simulink model "single_joint_controller_only"  (R2023b)
settings: Solver=FixedStepDiscrete  StartTime=0.0  StopTime=1.0  FixedStep=0.001  RelTol=1e-3
settings Model: Creator=user  LastModifiedBy=user
settings HardwareCC: ProdBitPerLong=64  ProdHWDeviceType=Intel->x86-64 (Linux 64)  TargetBitPerLong=64  TargetBitPerPointer=64  TargetBitPerSizeT=64  TargetBitPerPtrDiffT=64  TargetLargestAtomicFloat=Float  TargetIntDivRoundTo=Zero  TargetEndianess=LittleEndian  TargetWordSize=64  TargetHWDeviceType=Intel->x86-64 (Linux 64)  ProdEqTarget=off
settings RTWCC: GenerateReport=on

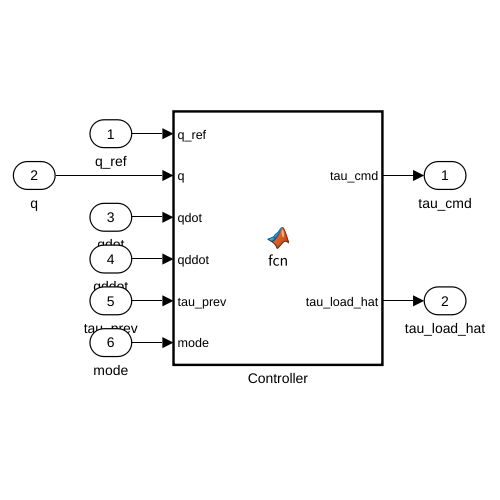
[thumbnail: Simulink's stored preview of the top-level diagram]
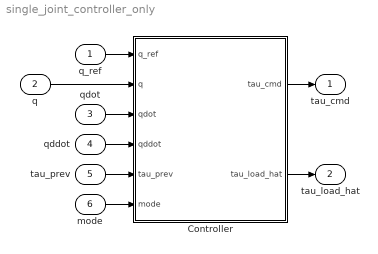
== system single_joint_controller_only ==
  q_ref : Inport  OutDataTypeStr=T_angle
  q : Inport  Port=2  OutDataTypeStr=T_angle
  qdot : Inport  Port=3  OutDataTypeStr=T_speed
  qddot : Inport  Port=4  OutDataTypeStr=T_accel
  tau_prev : Inport  Port=5  OutDataTypeStr=T_torque_wide
  mode : Inport  Port=6  OutDataTypeStr=uint8
  Controller : MATLAB Function  TreatAsAtomicUnit=on  RTWFcnName=usr_pid  RTWFileName=usr_pid
      settings: RTWFileNameOpts=User specified
  tau_cmd : Outport  OutDataTypeStr=T_torque
  tau_load_hat : Outport  Port=2  OutDataTypeStr=T_torque
  wires:
  q_ref/1 -> Controller/1(q_ref)
  q/1 -> Controller/2(q)
  qdot/1 -> Controller/3(qdot)
  qddot/1 -> Controller/4(qddot)
  tau_prev/1 -> Controller/5(tau_prev)
  mode/1 -> Controller/6(mode)
  Controller/1(tau_cmd) -> tau_cmd/1
  Controller/2(tau_load_hat) -> tau_load_hat/1

== matlab function single_joint_controller_only/Controller ==
  data: q_ref input; tau_cmd output; q input; qdot input; qddot input; tau_prev input; mode input; tau_load_hat output
function [tau_cmd, tau_load_hat] = fcn(q_ref, q, qdot, qddot, tau_prev, mode)
%#codegen
persistent integral_e dob_hat
if isempty(integral_e)
    integral_e = fi(0, 1, 16, 13);
    dob_hat = fi(0, 1, 16, 13);
end
q_ref_f = fi(q_ref, 1, 16, 12);
q_f = fi(q, 1, 16, 12);
qdot_f = fi(qdot, 1, 16, 8);
qddot_f = fi(qddot, 1, 16, 4);
tau_prev_f = fi(tau_prev, 1, 16, 12);
Ts = fi(0.001, 1, 16, 15);
tau_limit = fi(1.5, 1, 16, 13);
integral_limit = fi(0.40000000000000002, 1, 16, 13);
tau_hat_limit = fi(0.80000000000000004, 1, 16, 13);
Kp_pid = fi(8, 1, 16, 10);
Ki_pid = fi(6, 1, 16, 10);
Kd_pid = fi(0.45000000000000001, 1, 16, 14);
Kp_dob = fi(8, 1, 16, 10);
Kd_dob = fi(0.45000000000000001, 1, 16, 14);
Jn_dob = fi(0.01, 1, 16, 15);
bn_dob = fi(0.02, 1, 16, 15);
alpha_dob = fi(0.19741016454517191, 1, 16, 14);
K_imp = fi(4, 1, 16, 10);
D_imp = fi(0.38, 1, 16, 14);
e = fi(q_ref_f - q_f, 1, 16, 12);
tau_cmd = fi(0, 1, 16, 13);
tau_load_hat = fi(0, 1, 16, 13);
if mode < uint8(2)
    integral_e = fi(integral_e + Ts*e, 1, 16, 13);
    if integral_e > integral_limit
        integral_e = integral_limit;
    elseif integral_e < -integral_limit
        integral_e = -integral_limit;
    end
    tau_cmd = fi(Kp_pid*e + Ki_pid*integral_e - Kd_pid*qdot_f, 1, 16, 13);
elseif mode < uint8(3)
    raw_load = fi(tau_prev_f - Jn_dob*qddot_f - bn_dob*qdot_f, 1, 16, 13);
    dob_hat = fi(dob_hat + alpha_dob*(raw_load - dob_hat), 1, 16, 13);
    if dob_hat > tau_hat_limit
        dob_hat = tau_hat_limit;
    elseif dob_hat < -tau_hat_limit
        dob_hat = -tau_hat_limit;
    end
    tau_load_hat = dob_hat;
    tau_cmd = fi(Kp_dob*e - Kd_dob*qdot_f + tau_load_hat, 1, 16, 13);
else
    tau_cmd = fi(K_imp*e - D_imp*qdot_f, 1, 16, 13);
end
if tau_cmd > tau_limit
    tau_cmd = tau_limit;
elseif tau_cmd < -tau_limit
    tau_cmd = -tau_limit;
end
end
